simulink model "motorS22"  (R2022a)
settings: Solver=ode4  StartTime=0.0  StopTime=inf  FixedStep=0.001  RelTol=1e-3  EnableMultiTasking=on
model workspace (MAT data in the model file):
  Error = 0
libraries: arduinolib x6, simulink x2
settings Model: SimulationMode=external  ExtModeTrigDuration=2  Creator=Ninad  LastModifiedBy=deebarmaly
settings SolverCC: AlgebraicLoopSolver=TrustRegion
settings DataIOCC: LimitDataPoints=on  SaveFormat=Array  SignalLoggingSaveFormat=ModelDataLogs  ReturnWorkspaceOutputs=off
settings OptimizationCC: BlockReduction=off  EnhancedBackFolding=on  PassReuseOutputArgsThreshold=0  ExpressionDepthLimit=2147483647  MaxStackSize=64  OptimizeBlockOrder=speed  DifferentSizesBufferReuse=on  OptimizationCustomize=off
settings DebuggingCC: UnderspecifiedInitializationDetection=Classic  MergeDetectMultiDrivingBlocksExec=none  SolverPrmCheckMsg=warning  ParameterTunabilityLossMsg=error  FcnCallInpInsideContextMsg=warning  UnconnectedInputMsg=warning  UnconnectedOutputMsg=warning  UnconnectedLineMsg=warning  StateNameClashWarn=warning  SFUnexpectedBacktrackingDiag=warning  SFNoUnconditionalDefaultTransitionDiag=warning  SFExecutionAtInitializationDiag=none  SFMachineParentedDataDiag=warning  ArithmeticOperatorsInVariantConditions=warning
settings HardwareCC: ProdBitPerInt=16  ProdBitPerPointer=16  ProdBitPerSizeT=16  ProdBitPerPtrDiffT=16  ProdLargestAtomicFloat=None  ProdWordSize=8  ProdHWDeviceType=Atmel->AVR  UseEmbeddedCoderFeatures=off  UseSimulinkCoderFeatures=off
settings ModelReferenceCC: PropagateSignalLabelsOutOfModel=off
settings SFSimCC: SimUseLocalCustomCode=off  MATLABDynamicMemAlloc=off  CustomCodeUndefinedFunction=UseInterfaceOnly
settings RTWCC: SystemTargetFile=ert.tlc  HardwareBoard=Arduino Mega 2560  TemplateMakefile=ert_default_tmf  RTWUseLocalCustomCode=off  Toolchain=Arduino AVR  BuildConfiguration=Faster Runs  DLArmComputeVersion=19.05
settings CodeAppCC: ForceParamTrailComments=on  OperatorAnnotations=on
settings ERTTargetCC: ERTCustomFileBanners=off  SupportContinuousTime=on  SupportNonInlinedSFcns=on  RemoveResetFunc=off  SupportVariableSizeSignals=on  ModelStepFunctionPrototypeControlCompliant=off  ExtModeTransport=3  ExtModeStaticAlloc=on  ExtModeStaticAllocSize=2048  ExtModeMexFile=ext_xcp  ExtModeIntrfLevel=Level2 - Open  ERTSrcFileBannerTemplate=codertarget_code_template.cgt  ERTHdrFileBannerTemplate=codertarget_code_template.cgt  ERTDataSrcFileTemplate=codertarget_code_template.cgt  ERTDataHdrFileTemplate=codertarget_code_template.cgt
settings ConfigComp: CovMetricSettings=dw  CovSaveCumulativeToWorkspaceVar=on  CovSaveSingleToWorkspaceVar=on  CovExternalEMLEnable=off  CovSFcnEnable=off

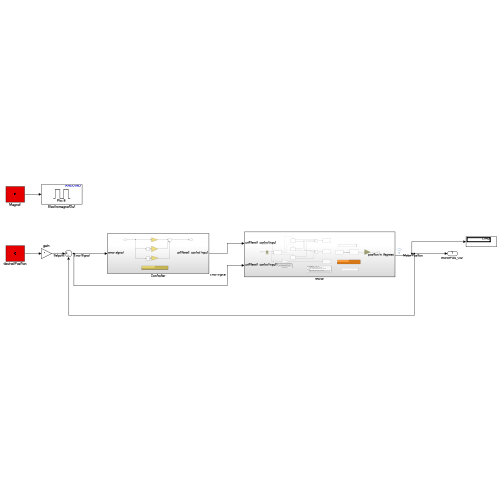
[thumbnail: Simulink's stored preview of the top-level diagram]
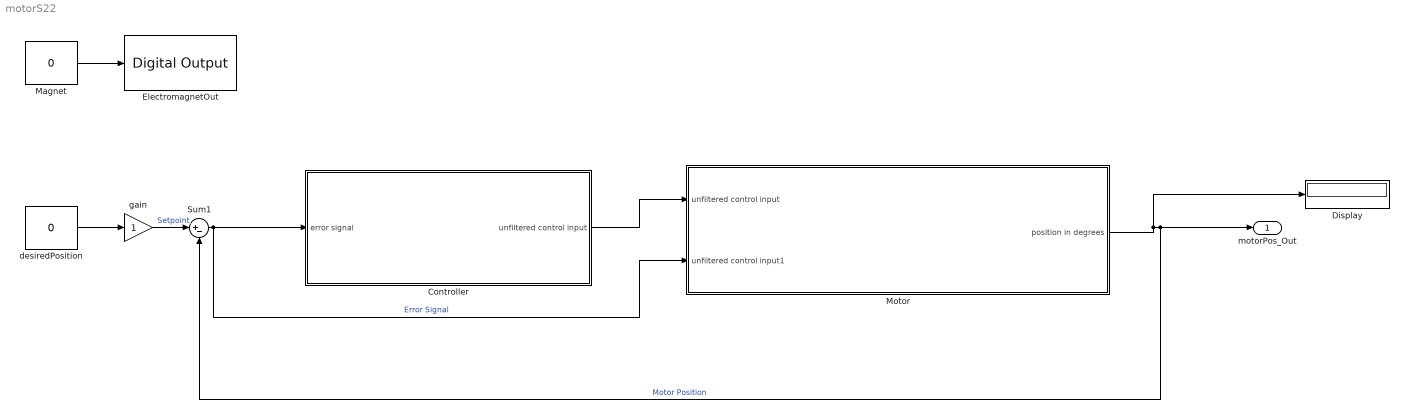
== system motorS22 ==
  Controller : Subsystem
  Display : Display
  ElectromagnetOut : arduinolib/Digital Output  pinNumber=8  Direction=output  blockPlatform=arduino
  Magnet : Constant  Value=0
  Motor : Subsystem
  Sum1 : Sum  Inputs=|+-
  desiredPosition : Constant  Value=0
  gain : Gain
  motorPos_Out : Outport  VectorParamsAs1DForOutWhenUnconnected=off
  wires:
  gain/1 -> Sum1/1  "Setpoint"
  Motor/1(position in degrees) -> Sum1/2, motorPos_Out/1, Display/1  "Motor Position"
  Controller/1(unfiltered control input) -> Motor/1(unfiltered control input)
  Sum1/1 -> Motor/2(unfiltered control input1), Controller/1(error signal)  "Error Signal"
  desiredPosition/1 -> gain/1
  Magnet/1 -> ElectromagnetOut/1

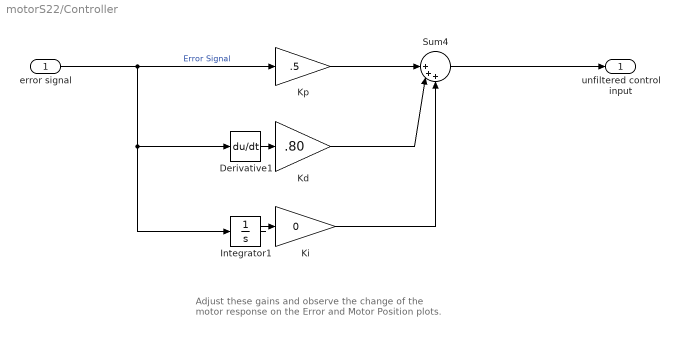
== system motorS22/Controller ==
  note: Adjust these gains and observe the change of the
      | motor response on the Error and Motor Position
      | plots.
  error signal : Inport
  Derivative1 : Derivative
  Integrator1 : Integrator
  Kd : Gain  Gain=.80
  Ki : Gain  Gain=0
  Kp : Gain  Gain=.5
  Sum4 : Sum  Inputs=||+++
  unfiltered control input : Outport
  wires:
  Kd/1 -> Sum4/2
  Integrator1/1 -> Ki/1
  Ki/1 -> Sum4/3
  Derivative1/1 -> Kd/1
  error signal/1 -> Derivative1/1, Integrator1/1, Kp/1  "Error Signal"
  Kp/1 -> Sum4/1
  Sum4/1 -> unfiltered control input/1

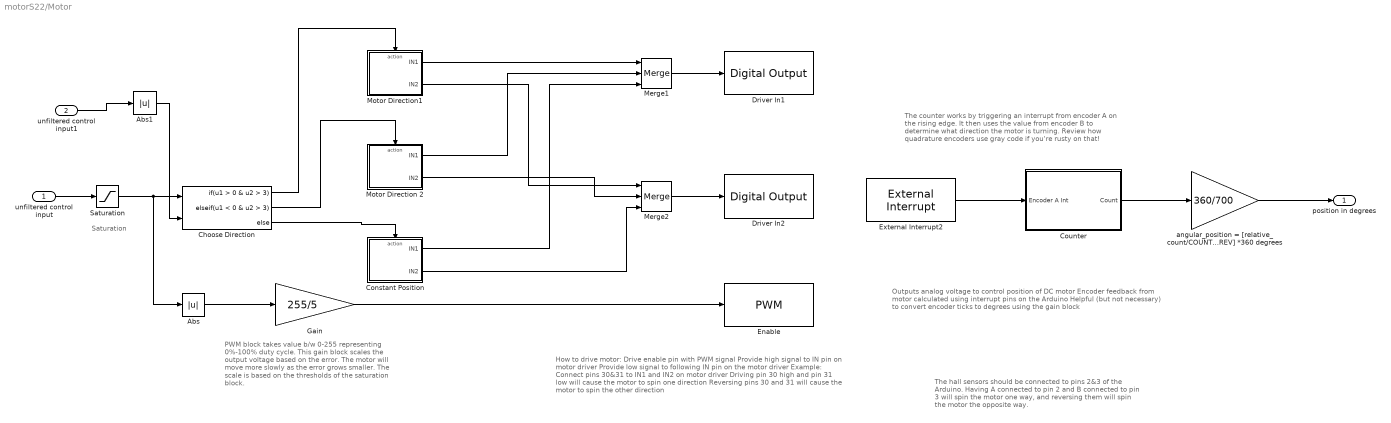
== system motorS22/Motor ==
  note: The counter works by triggering an interrupt from encoder A
      | on the rising edge. It then uses the value from encoder B to
      | determine what direction the motor is turning. Review how
      | quadrature encoders use gray code if you're rusty on that!
  note: PWM block takes value b/w 0-255 representing
      | 0%-100% duty cycle. This gain block scales the
      | output voltage based on the error. The motor will
      | move more slowly as the error grows
      | smaller. The scale is based on the thresholds
      | of the saturation block.
  note: Outputs analog voltage to control position of DC motor
      |
      | Encoder feedback from motor calculated using interrupt pins on the Arduino
      |
      | Helpful (but not necessary) to convert encoder ticks to degrees using the
      | gain block
  note: Saturation
  note: How to drive motor:
      | Drive enable pin with PWM signal
      | Provide high signal to IN pin on motor driver
      | Provide low signal to following IN pin on the motor driver
      |
      | Example:
      | Connect pins 30&31 to IN1 and IN2 on motor driver
      | Driving pin 30 high and pin 31 low will cause the motor to spin one direction
      | Reversing pins 30 and 31 will cause the motor to spin the other direction
  note: The hall sensors should be connected to pins 2&3 of the
      | Arduino. Having A connected to pin 2 and B connected to
      | pin 3 will spin the motor one way, and reversing them will
      | spin the motor the opposite way.
  unfiltered control input : Inport
  unfiltered control input1 : Inport  Port=2
  Abs : Abs  SaturateOnIntegerOverflow=off
  Abs1 : Abs  SaturateOnIntegerOverflow=off
  Choose Direction : If  NumInputs=2  IfExpression=u1 > 0 & u2 > 3  ElseIfExpressions=u1 < 0 & u2 > 3
  Constant Position : Subsystem  TreatAsAtomicUnit=on
  Counter : Subsystem
  Driver In1 : arduinolib/Digital Output  pinNumber=30  Direction=output  blockPlatform=arduino
  Driver In2 : arduinolib/Digital Output  pinNumber=31  Direction=output  blockPlatform=arduino
  Enable : arduinolib/PWM  pinNumber=5  frequencyType=Default  desiredFrequency=490.2  achievableFrequency=490.2
  External Interrupt2 : arduinolib/External Interrupt  Pin=2  PullUp=on  Mode=RISING  InterruptSimulationInput=off
      settings: SourceProductBaseCode=ARDUINO
  Gain : Gain  Gain=255/5
  Merge1 : Merge  Inputs=3
  Merge2 : Merge  Inputs=3
  Motor Direction 2 : Subsystem  TreatAsAtomicUnit=on
  Motor Direction1 : Subsystem  TreatAsAtomicUnit=on
  Saturation : Saturate  UpperLimit=5  LowerLimit=-5
  angular_position = [relative_count/COUNTS_PER_REV] *360 degrees : Gain  Gain=360/700
  position in degrees : Outport  VectorParamsAs1DForOutWhenUnconnected=off
  wires:
  angular_position = [relative_count/COUNTS_PER_REV] *360 degrees/1 -> position in degrees/1
  unfiltered control input/1 -> Saturation/1
  Counter/1(Count) -> angular_position = [relative_count/COUNTS_PER_REV] *360 degrees/1
  Saturation/1 -> Abs/1, Choose Direction/1
  Choose Direction/1 -> Motor Direction1/Action
  Motor Direction1/1(IN1) -> Merge1/1
  Motor Direction 2/1(IN1) -> Merge1/2
  Motor Direction1/2(IN2) -> Merge2/1
  Motor Direction 2/2(IN2) -> Merge2/2
  Abs/1 -> Gain/1
  Gain/1 -> Enable/1
  Merge1/1 -> Driver In1/1
  Merge2/1 -> Driver In2/1
  External Interrupt2/1 -> Counter/1(Encoder A Int)
  Constant Position/2(IN2) -> Merge2/3
  Constant Position/1(IN1) -> Merge1/3
  unfiltered control input1/1 -> Abs1/1
  Abs1/1 -> Choose Direction/2
  Choose Direction/3 -> Constant Position/Action
  Choose Direction/2 -> Motor Direction 2/Action

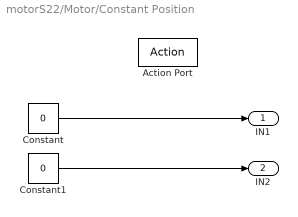
== system motorS22/Motor/Constant Position ==
  Action Port : ActionPort  ActionPortLabel=else
  Constant : Constant  Value=0
  Constant1 : Constant  Value=0
  IN1 : Outport
  IN2 : Outport  Port=2
  wires:
  Constant/1 -> IN1/1
  Constant1/1 -> IN2/1

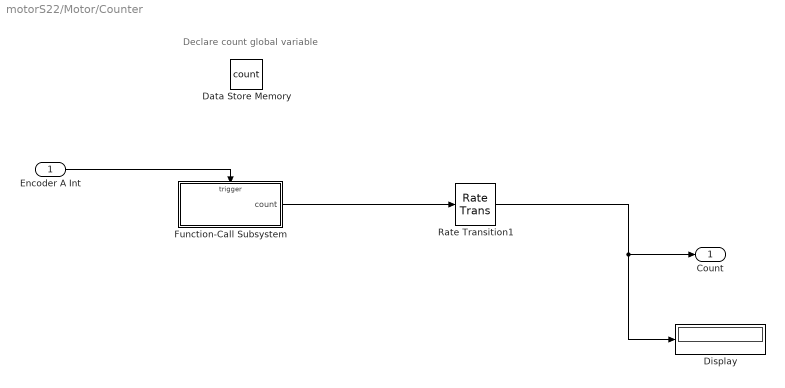
== system motorS22/Motor/Counter ==
  note: Declare count global variable
  Encoder A Int : Inport
  Data Store Memory : DataStoreMemory  DataStoreName=count  ReadBeforeWriteMsg=warning  WriteAfterWriteMsg=warning  WriteAfterReadMsg=warning  ShowAdditionalParam=off
  Display : Display
  Function-Call Subsystem : Subsystem  TreatAsAtomicUnit=on
  Rate Transition1 : RateTransition  Deterministic=off
  Count : Outport
  wires:
  Encoder A Int/1 -> Function-Call Subsystem/Trigger
  Function-Call Subsystem/1(count) -> Rate Transition1/1
  Rate Transition1/1 -> Display/1, Count/1

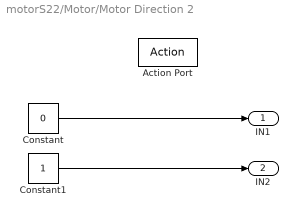
== system motorS22/Motor/Motor Direction 2 ==
  Action Port : ActionPort  ActionPortLabel=elseif(u1 < 0 & u2 > 3)
  Constant : Constant  Value=0
  Constant1 : Constant
  IN1 : Outport
  IN2 : Outport  Port=2
  wires:
  Constant/1 -> IN1/1
  Constant1/1 -> IN2/1

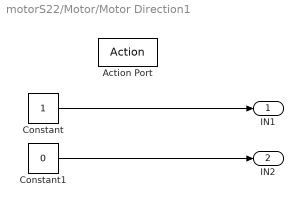
== system motorS22/Motor/Motor Direction1 ==
  Action Port : ActionPort  ActionPortLabel=if(u1 > 0 & u2 > 3)
  Constant : Constant
  Constant1 : Constant  Value=0
  IN1 : Outport
  IN2 : Outport  Port=2
  wires:
  Constant/1 -> IN1/1
  Constant1/1 -> IN2/1

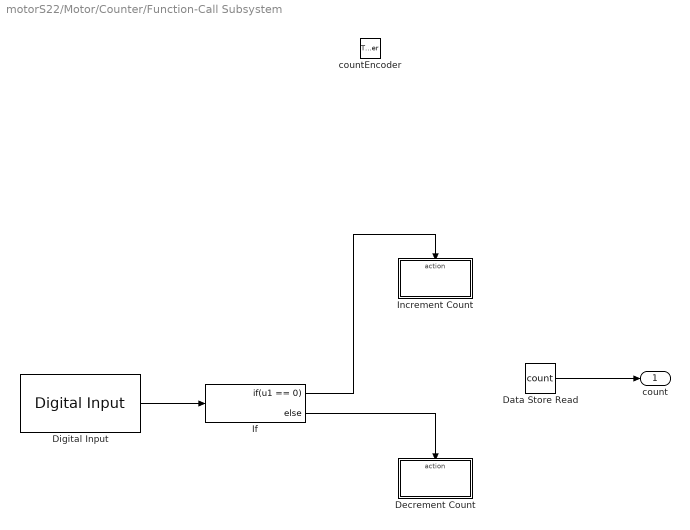
== system motorS22/Motor/Counter/Function-Call Subsystem ==
  countEncoder : TriggerPort  TriggerType=function-call  VariantControl=Variant
  Data Store Read : DataStoreRead  DataStoreName=count  IndexOptions=Index vector (dialog)  Indices=1  OutputSizes=1
  Decrement Count : Subsystem  TreatAsAtomicUnit=on
  Digital Input : arduinolib/Digital Input  pinNumber=3  mode=Default  Direction=input  SampleTime=-1  blockPlatform=arduino
  If : If  IfExpression=u1 == 0
  Increment Count : Subsystem  TreatAsAtomicUnit=on
  count : Outport
  wires:
  If/2 -> Decrement Count/Action
  If/1 -> Increment Count/Action
  Data Store Read/1 -> count/1
  Digital Input/1 -> If/1

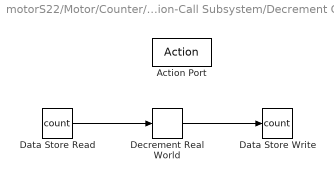
== system motorS22/Motor/Counter/Function-Call Subsystem/Decrement Count ==
  Action Port : ActionPort  ActionPortLabel=else
  Data Store Read : DataStoreRead  DataStoreName=count  IndexOptions=Index vector (dialog)  Indices=1  OutputSizes=1
  Data Store Write : DataStoreWrite  DataStoreName=count  IndexOptions=Index vector (dialog)  Indices=1  OutputSizes=1
  Decrement Real World : simulink/Additional Math & Discrete/Additional Math: Increment - Decrement/Decrement Real World
      settings: SourceProductBaseCode=SL
  wires:
  Data Store Read/1 -> Decrement Real World/1
  Decrement Real World/1 -> Data Store Write/1

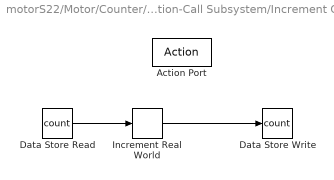
== system motorS22/Motor/Counter/Function-Call Subsystem/Increment Count ==
  Action Port : ActionPort  ActionPortLabel=if(u1 == 0)
  Data Store Read : DataStoreRead  DataStoreName=count  IndexOptions=Index vector (dialog)  Indices=1  OutputSizes=1
  Data Store Write : DataStoreWrite  DataStoreName=count  IndexOptions=Index vector (dialog)  Indices=1  OutputSizes=1
  Increment Real World : simulink/Additional Math & Discrete/Additional Math: Increment - Decrement/Increment Real World
      settings: SourceProductBaseCode=SL
  wires:
  Data Store Read/1 -> Increment Real World/1
  Increment Real World/1 -> Data Store Write/1
